simulink model "model_wszystkie_3"  (R2024a)
settings: Solver=ode45  StartTime=0.0  StopTime=60  RelTol=1e-3
InitFcn:
  | a = 0.672; % M + ma/2 + mb, kg
  | b = 0.0051; % (ma/2 + mb)*L, kg*m
  | % c = 0.0021; % (ma/4 + mb)*L^2 + I, kg*m^2
  | g = 9.81;
  | u = 1;
  | 
  | T1 = 0.2;
  | T2 = 0.1;
  | Tf = 0.05;
  | 
  | x1 = 0;
  | x2 = 0;
  | x3 = 0;
  | x4 = 0;
  | x1p = 0;
  | x2p = 0;
  | x3p = 0;
  | x4p = 0;
  | 
  | r = 1;
  | 
  | b0 = 1;
  | A = [0 1 0;
  |      0 0 1;
  |      0 0 0];
  | b_ = [0; b0; 0];
  | c = [1; 0; 0];
  | 
  | % A_CP = [0 1;
  | %        0 0];
  | %
  | % b_CP = [0; 1];
  | %
  | % w_CL = 70;
  | %
  | % k = place(A_CP', b_CP, -w_CL*[1 1.01])';
  | %
  | % k_ESO = 0.9;
  | %
  | % l = place(A',c,-w_CL*k_ESO*[0.99,1,1.01])';
  | 
  | % k_ESO = 10;
  | 
  | % wc_ = 70;
  | % Kx_ = place(A',b_,-wc_*[1 1])';
  | %
  | % k = [5;5];
  | %
  | % w0 = 60;
  | % l = place(A',c,-w0*[0.99,1,1.01])';
  | 
  | %% Liczenie k
  | w_CL = 5;
  | n=2;
  | k = zeros(n,1);
  | for i = 1:n
  |     k(i) = ((factorial(n))/(factorial(n-i+1)*factorial(i-1)))*w_CL^(n-i+1);
  | end
  | 
  | k_r = [k(2); 1];
  | 
  | %% Liczenie l
  | k_ESO = 50;
  | l = zeros(n+1,1);
  | 
  | for i = 1:n+1
  |     l(i) = (factorial(n+1)/(factorial(n-i+1)*factorial(i)))*(k_ESO)^(i);
  | end
  | 
  | % %% PRZYPISANIE POSZCZEGÓLNYCH L:
  | % l1 = l(1);
  | % l2 = l(2);
  | % %% OKREŚLENIE BETY:
  | % B1 = 3 * k_ESO;
  | % B2 = 3 * k_ESO^2;
  | % B3 = k_ESO^3;
  | 
  | %% W ARTYKULE MADONSKI K,L ODPOWIADA L I B W ARTYKULE JIN H.
  | l1 = k(2);
  | l2 = k(1);
  | 
  | B1 = l(1);
  | B2 = l(2);
  | B3 = l(3);
  | 
  | %% WYZNACZENIE PARAMETRÓW:
  | Kc = (B2 * l2 + B3 * l1)/(b0*(B1 * l1 + B2 + l2));
  | tau_i = (B2 * l2 + B3 * l1)/(B3 * l2);
  | tau_d = (B1 * l2 + B2 * l1 + B3)/(B2 * l2 + B3 * l1);
  | wl = sqrt(B1 * l1 + B2 + l2);
  | zeta_l = (B1 + l1)/(2*sqrt(B1 * l1 + B2 + l2));
  | %% Wzmocnienia regulatora CPID:
  | Kp = Kc;
  | Ki = Kc/tau_i;
  | Kd = Kc * tau_d;
  | 
  | %% NOWE NASTAWY PID
  | % Kp = (k(1)*l(1)+k(2)*l(3))/(b0*(k(2)*l(1)+l(2)+k(1)));
  | % Ki = (k(1)*l(3))/(b0*(k(2)*l(1)+l(2)+k(1)));
  | % Kd = (k(1)*l(1)+k(2)*l(2)+l(3))/(b0*(k(2)*l(1)+l(2)+k(1)));
libraries: simulink x4, slpidlib x1
settings Model: Creator=kubat  LastModifiedBy=kubat
settings OptimizationCC: ReuseModelBlockBuffer=off
settings RTWCC: GPUComputeCapability=3.5

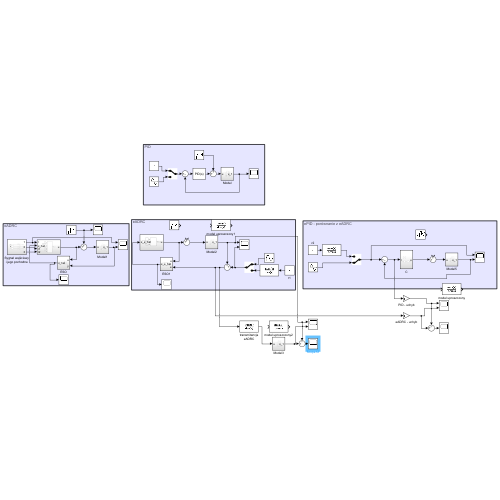
[thumbnail: Simulink's stored preview of the top-level diagram]
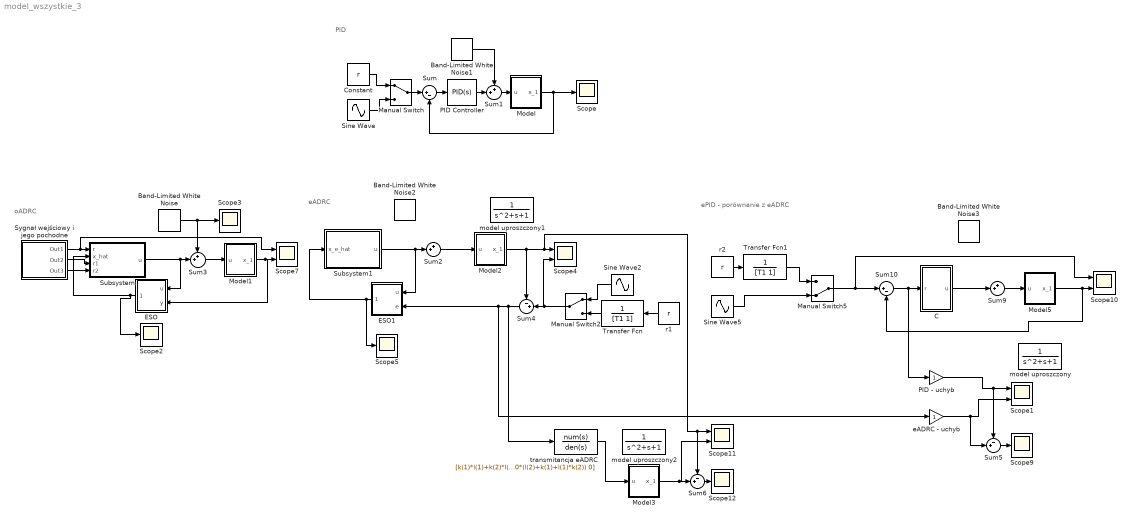
== system model_wszystkie_3 ==
  note: eADRC
  note: oADRC
  note: PID
  note: ePID - porównanie z eADRC
  Band-Limited White Noise{,1..3} (4 alike) : simulink/Sources/Band-Limited White Noise  Cov=[0.001]  Ts=0.01  seed=[23341]
  C : Subsystem
  Constant : Constant  Value=r
  ESO : Subsystem
  ESO1 : Subsystem
  Manual Switch : ManualSwitch
  Manual Switch2 : ManualSwitch
  Manual Switch5 : ManualSwitch  CurrentSetting=0
  Model : Subsystem
  Model1 : Subsystem
  Model2 : Subsystem
  Model3 : Subsystem
  Model5 : Subsystem
  PID - uchyb : Gain
  PID Controller : slpidlib/PID Controller  Controller=PID  Form=Parallel  TimeDomain=Continuous-time  UseExternalTs=off  SampleTime=-1  IntegratorMethod=Forward Euler  FilterMethod=Forward Euler  ControllerParametersSource=internal  P=0.00659119654590323  I=2.38451819654017e-05  UseKiTs=off  D=0.404807783978182  UseExternalDerivativeSource=off  N=70.8689683200542  UseFilter=on  TunerSelectOption=Transfer Function Based (PID Tuner App)  InitialConditionSource=internal  InitialConditionForIntegrator=0  InitialConditionForFilter=0  DifferentiatorICPrevScaledInput=0  ExternalReset=none  TrackingMode=off  Kt=1  LimitOutput=off  SatLimitsSource=internal  UpperSaturationLimit=inf  LowerSaturationLimit=-inf  LinearizeAsGain=on  AntiWindupMode=none  Kb=1  LimitIntegrator=off  UpperIntegratorSaturationLimit=inf  LowerIntegratorSaturationLimit=-inf  POutMin=[]  POutMax=[]  IOutMin=[]  IOutMax=[]  DOutMin=[]  DOutMax=[]  NOutMin=[]  NOutMax=[]  SumOutMin=[]  SumOutMax=[]  SaturationOutMin=[]  SaturationOutMax=[]  PParamMin=[]  PParamMax=[]  IParamMin=[]  IParamMax=[]  DParamMin=[]  DParamMax=[]  NParamMin=[]  NParamMax=[]  KbParamMin=[]  KbParamMax=[]  KtParamMin=[]  KtParamMax=[]  KbOutMin=[]  KbOutMax=[]  KtOutMin=[]  KtOutMax=[]  IntegratorOutMin=[]  IntegratorOutMax=[]  FilterOutMin=[]  FilterOutMax=[]  SumI1OutMin=[]  SumI1OutMax=[]  SumI2OutMin=[]  SumI2OutMax=[]  SumI3OutMin=[]  SumI3OutMax=[]  SumI4OutMin=[]  SumI4OutMax=[]  SumDOutMin=[]  SumDOutMax=[]  DifferentiatorOutMin=[]  DifferentiatorOutMax=[]  FilterDiffOutCoefMin=[]  FilterDiffOutCoefMax=[]  ReciprocalOutMin=[]  ReciprocalOutMax=[]  SumDenOutMin=[]  SumDenOutMax=[]  SumNumOutMin=[]  SumNumOutMax=[]  DivideOutMin=[]  DivideOutMax=[]  UdiffTsProdOutMin=[]  UdiffTsProdOutMax=[]  NTsProdOutMin=[]  NTsProdOutMax=[]  UintegralTsProdOutMin=[]  UintegralTsProdOutMax=[]  UngainTsProdOutMin=[]  UngainTsProdOutMax=[]  ClampingZeroOutDataTypeStr=Inherit: Inherit via back propagation  ClampingZeroOutMin=[]  ClampingZeroOutMax=[]  FilterDenConstantOutDataTypeStr=Inherit: Inherit via back propagation  FilterDenConstantOutMin=[]  FilterDenConstantOutMax=[]  PCopyOutDataTypeStr=Inherit: Inherit via back propagation  PCopyOutMin=[]  PCopyOutMax=[]  NCopyOutDataTypeStr=Inherit: Inherit via back propagation  NCopyOutMin=[]  NCopyOutMax=[]  IntegratorContinuousStateAttributes=''  IntegratorStateMustResolveToSignalObject=off  IntegratorRTWStateStorageClass=Auto  FilterContinuousStateAttributes=''  FilterStateMustResolveToSignalObject=off  FilterRTWStateStorageClass=Auto  ParallelPVariant=InternalParameters  IdealPVariant=Disabled  IVariant=InternalParameters  DVariant=InternalParameters  IntegratorVariant=Continuous  SatVariant=Disabled  AWVariant=Passthrough  PCopyVariant=Disabled  TRVariant=Disabled  FdbkBlocksVariant=Forward  IdealPFdbkVariant=Disabled  SatFdbkVariant=Disabled  DerivativeFilterVariant=ContFilter  NVariant=InternalParameters  NCopyVariant=Disabled  FilterICVariant=InternalICsFilter  IntegratorICVariant=InternalICs  ExternalResetVariant=Disabled  TRSumVariant=Passthrough  SumFdbkVariant=Disabled  SumVariant=Sum_PID  TsampFilterVariant=InternalTs  TsampNgainVariant=Passthrough  TsampIntegralVariant=Disabled_SignalSpec  ExternalSaturationOutDataTypeStr=Inherit: Same as second input  DerivativeSourceVariant=ErrorSignal
  Scope{,2..3,5,9,12} (6 alike) : Scope
  Scope{1,4,7,10..11} (5 alike) : Scope  NumInputPorts=2
  Sine Wave : Sin  Amplitude=u  SampleTime=0
  Sine Wave2 : Sin  Amplitude=u  SampleTime=0
  Sine Wave5 : Sin  Amplitude=u  SampleTime=0
  Subsystem : Subsystem
  Subsystem1 : Subsystem
  Sum : Sum  Inputs=|+-
  Sum{1..3,9} (4 alike) : Sum  Inputs=++|
  Sum10 : Sum  Inputs=|+-
  Sum4 : Sum  Inputs=-+|
  Sum5 : Sum  Inputs=-+|
  Sum6 : Sum  Inputs=-+|
  Sygnał wejściowy i jego pochodne : Subsystem
  Transfer Fcn : TransferFcn  Denominator=[T1 1]
  Transfer Fcn1 : TransferFcn  Denominator=[T1 1]
  eADRC - uchyb : Gain
  model uproszczony : TransferFcn  Denominator=[1 1 1]
  model uproszczony1 : TransferFcn  Denominator=[1 1 1]
  model uproszczony2 : TransferFcn  Denominator=[1 1 1]
  r1 : Constant  Value=r
  r2 : Constant  Value=r
  transmitancja eADRC : TransferFcn  Numerator=[k(1)*l(1)+k(2)*l(2)+l(3) k(1)*l(2)+k(2)*l(3) k(1)*l(3)]  Denominator=[b0 b0*(k(2)+l(1)) b0*(l(2)+k(1)+l(1)*k(2)) 0]
  wires:
  Model/1(x_1) -> Scope/1, Sum/2
  Sum/1 -> PID Controller/1
  Manual Switch/1 -> Sum/1
  Constant/1 -> Manual Switch/1
  Sine Wave/1 -> Manual Switch/2
  Model1/1(x_1) -> ESO/2(y), Scope7/2
  Sum3/1 -> Model1/1(u)
  Subsystem/1(u) -> ESO/1(u), Sum3/2
  ESO/1(x_hat) -> Scope2/1, Subsystem/2(x_hat)
  Band-Limited White Noise/1 -> Sum3/1, Scope3/1
  PID Controller/1 -> Sum1/2
  Sum1/1 -> Model/1(u)
  Band-Limited White Noise1/1 -> Sum1/1
  ESO1/1(x_e_hat) -> Subsystem1/1(x_e_hat), Scope5/1
  Subsystem1/1(u) -> ESO1/1(u), Sum2/2
  Sum4/1 -> transmitancja eADRC/1, eADRC - uchyb/1, ESO1/2(e)
  Sine Wave2/1 -> Manual Switch2/1
  Manual Switch2/1 -> Scope4/2, Sum4/2
  Transfer Fcn/1 -> Manual Switch2/2
  r1/1 -> Transfer Fcn/1
  Sygnał wejściowy i jego pochodne/1(Out1) -> Scope7/1, Subsystem/1(r)
  Sygnał wejściowy i jego pochodne/2(Out2) -> Subsystem/3(r1)
  Sygnał wejściowy i jego pochodne/3(Out3) -> Subsystem/4(r2)
  C/1(u) -> Sum9/2
  Sum10/1 -> PID - uchyb/1, C/1(r)
  Sine Wave5/1 -> Manual Switch5/2
  Manual Switch5/1 -> Scope10/1, Sum10/1
  Transfer Fcn1/1 -> Manual Switch5/1
  r2/1 -> Transfer Fcn1/1
  PID - uchyb/1 -> Sum5/1, Scope1/1
  eADRC - uchyb/1 -> Sum5/2, Scope1/2
  Sum5/1 -> Scope9/1
  Sum9/1 -> Model5/1(u)
  Model5/1(x_1) -> Sum10/2, Scope10/2
  Sum2/1 -> Model2/1(u)
  Model2/1(x_1) -> Scope11/1, Sum6/1, Scope4/1, Sum4/1
  transmitancja eADRC/1 -> Model3/1(u)
  Model3/1(x_1) -> Scope11/2, Sum6/2
  Sum6/1 -> Scope12/1

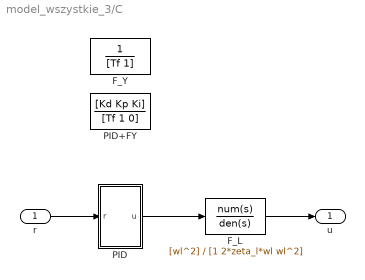
== system model_wszystkie_3/C ==
  r : Inport
  F_L : TransferFcn  Numerator=[wl^2]  Denominator=[1 2*zeta_l*wl wl^2]
  F_Y : TransferFcn  Denominator=[Tf 1]
  PID : Subsystem
  PID+FY : TransferFcn  Numerator=[Kd Kp Ki]  Denominator=[Tf 1 0]
  u : Outport
  wires:
  PID/1(u) -> F_L/1
  r/1 -> PID/1(r)
  F_L/1 -> u/1

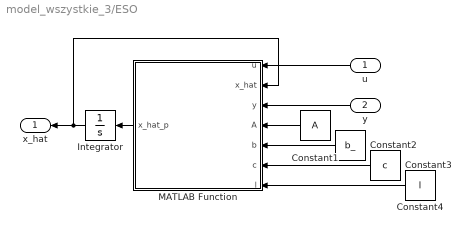
== system model_wszystkie_3/ESO ==
  u : Inport
  y : Inport  Port=2
  Constant1 : Constant  Value=A
  Constant2 : Constant  Value=b_
  Constant3 : Constant  Value=c
  Constant4 : Constant  Value=l
  Integrator : Integrator
  MATLAB Function : MATLAB Function  TreatAsAtomicUnit=on
  x_hat : Outport
  wires:
  Constant3/1 -> MATLAB Function/6(c)
  Integrator/1 -> x_hat/1, MATLAB Function/2(x_hat)
  MATLAB Function/1(x_hat_p) -> Integrator/1
  Constant2/1 -> MATLAB Function/5(b)
  y/1 -> MATLAB Function/3(y)
  Constant1/1 -> MATLAB Function/4(A)
  Constant4/1 -> MATLAB Function/7(l)
  u/1 -> MATLAB Function/1(u)

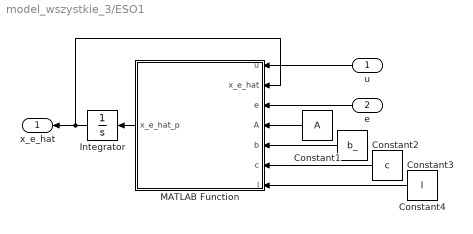
== system model_wszystkie_3/ESO1 ==
  u : Inport
  e : Inport  Port=2
  Constant1 : Constant  Value=A
  Constant2 : Constant  Value=b_
  Constant3 : Constant  Value=c
  Constant4 : Constant  Value=l
  Integrator : Integrator
  MATLAB Function : MATLAB Function  TreatAsAtomicUnit=on
  x_e_hat : Outport
  wires:
  Constant3/1 -> MATLAB Function/6(c)
  Integrator/1 -> x_e_hat/1, MATLAB Function/2(x_e_hat)
  MATLAB Function/1(x_e_hat_p) -> Integrator/1
  Constant2/1 -> MATLAB Function/5(b)
  e/1 -> MATLAB Function/3(e)
  Constant1/1 -> MATLAB Function/4(A)
  Constant4/1 -> MATLAB Function/7(l)
  u/1 -> MATLAB Function/1(u)

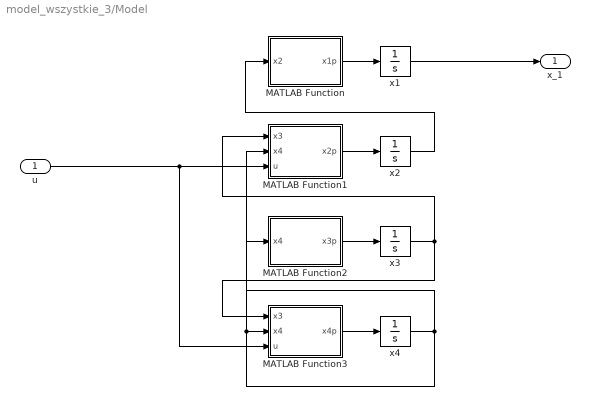
== system model_wszystkie_3/Model ==
  u : Inport
  MATLAB Function : MATLAB Function  TreatAsAtomicUnit=on
  MATLAB Function1 : MATLAB Function  TreatAsAtomicUnit=on
  MATLAB Function2 : MATLAB Function  TreatAsAtomicUnit=on
  MATLAB Function3 : MATLAB Function  TreatAsAtomicUnit=on
  x{1..4} (4 alike) : Integrator
  x_1 : Outport
  wires:
  u/1 -> MATLAB Function3/3(u), MATLAB Function1/3(u)
  x4/1 -> MATLAB Function3/2(x4), MATLAB Function1/2(x4), MATLAB Function2/1(x4)
  MATLAB Function/1(x1p) -> x1/1
  x3/1 -> MATLAB Function1/1(x3), MATLAB Function3/1(x3)
  x2/1 -> MATLAB Function/1(x2)
  MATLAB Function2/1(x3p) -> x3/1
  MATLAB Function1/1(x2p) -> x2/1
  MATLAB Function3/1(x4p) -> x4/1
  x1/1 -> x_1/1

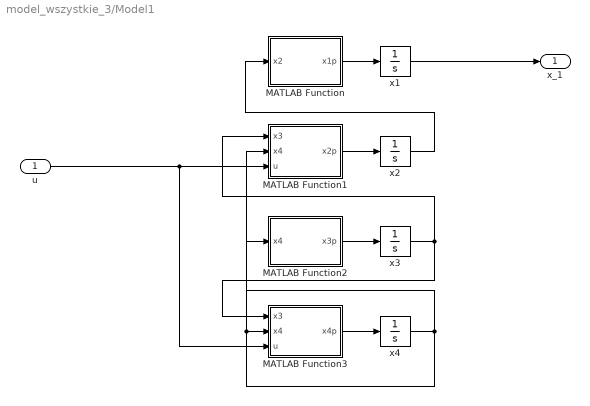
== system model_wszystkie_3/Model1 ==
  u : Inport
  MATLAB Function : MATLAB Function  TreatAsAtomicUnit=on
  MATLAB Function1 : MATLAB Function  TreatAsAtomicUnit=on
  MATLAB Function2 : MATLAB Function  TreatAsAtomicUnit=on
  MATLAB Function3 : MATLAB Function  TreatAsAtomicUnit=on
  x{1..4} (4 alike) : Integrator
  x_1 : Outport
  wires:
  u/1 -> MATLAB Function3/3(u), MATLAB Function1/3(u)
  x4/1 -> MATLAB Function3/2(x4), MATLAB Function1/2(x4), MATLAB Function2/1(x4)
  MATLAB Function/1(x1p) -> x1/1
  x3/1 -> MATLAB Function1/1(x3), MATLAB Function3/1(x3)
  x2/1 -> MATLAB Function/1(x2)
  MATLAB Function2/1(x3p) -> x3/1
  MATLAB Function1/1(x2p) -> x2/1
  MATLAB Function3/1(x4p) -> x4/1
  x1/1 -> x_1/1

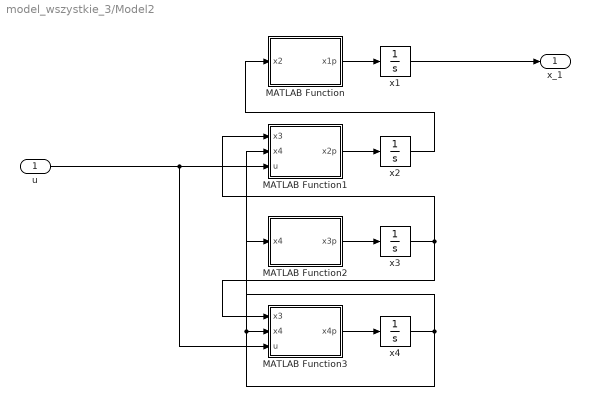
== system model_wszystkie_3/Model2 ==
  u : Inport
  MATLAB Function : MATLAB Function  TreatAsAtomicUnit=on
  MATLAB Function1 : MATLAB Function  TreatAsAtomicUnit=on
  MATLAB Function2 : MATLAB Function  TreatAsAtomicUnit=on
  MATLAB Function3 : MATLAB Function  TreatAsAtomicUnit=on
  x{1..4} (4 alike) : Integrator
  x_1 : Outport
  wires:
  u/1 -> MATLAB Function3/3(u), MATLAB Function1/3(u)
  x4/1 -> MATLAB Function2/1(x4), MATLAB Function3/2(x4), MATLAB Function1/2(x4)
  MATLAB Function/1(x1p) -> x1/1
  x3/1 -> MATLAB Function1/1(x3), MATLAB Function3/1(x3)
  x2/1 -> MATLAB Function/1(x2)
  MATLAB Function2/1(x3p) -> x3/1
  MATLAB Function1/1(x2p) -> x2/1
  MATLAB Function3/1(x4p) -> x4/1
  x1/1 -> x_1/1

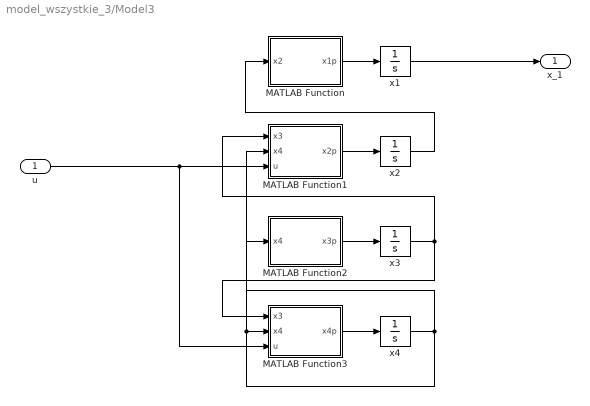
== system model_wszystkie_3/Model3 ==
  u : Inport
  MATLAB Function : MATLAB Function  TreatAsAtomicUnit=on
  MATLAB Function1 : MATLAB Function  TreatAsAtomicUnit=on
  MATLAB Function2 : MATLAB Function  TreatAsAtomicUnit=on
  MATLAB Function3 : MATLAB Function  TreatAsAtomicUnit=on
  x{1..4} (4 alike) : Integrator
  x_1 : Outport
  wires:
  u/1 -> MATLAB Function3/3(u), MATLAB Function1/3(u)
  x4/1 -> MATLAB Function3/2(x4), MATLAB Function1/2(x4), MATLAB Function2/1(x4)
  MATLAB Function/1(x1p) -> x1/1
  x3/1 -> MATLAB Function1/1(x3), MATLAB Function3/1(x3)
  x2/1 -> MATLAB Function/1(x2)
  MATLAB Function2/1(x3p) -> x3/1
  MATLAB Function1/1(x2p) -> x2/1
  MATLAB Function3/1(x4p) -> x4/1
  x1/1 -> x_1/1

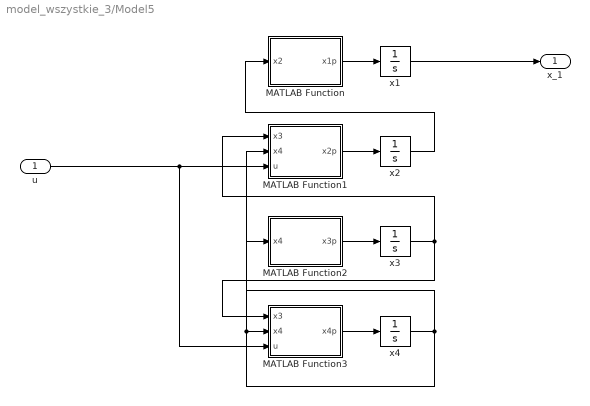
== system model_wszystkie_3/Model5 ==
  u : Inport
  MATLAB Function : MATLAB Function  TreatAsAtomicUnit=on
  MATLAB Function1 : MATLAB Function  TreatAsAtomicUnit=on
  MATLAB Function2 : MATLAB Function  TreatAsAtomicUnit=on
  MATLAB Function3 : MATLAB Function  TreatAsAtomicUnit=on
  x{1..4} (4 alike) : Integrator
  x_1 : Outport
  wires:
  u/1 -> MATLAB Function3/3(u), MATLAB Function1/3(u)
  x4/1 -> MATLAB Function3/2(x4), MATLAB Function1/2(x4), MATLAB Function2/1(x4)
  MATLAB Function/1(x1p) -> x1/1
  x3/1 -> MATLAB Function1/1(x3), MATLAB Function3/1(x3)
  x2/1 -> MATLAB Function/1(x2)
  MATLAB Function2/1(x3p) -> x3/1
  MATLAB Function1/1(x2p) -> x2/1
  MATLAB Function3/1(x4p) -> x4/1
  x1/1 -> x_1/1

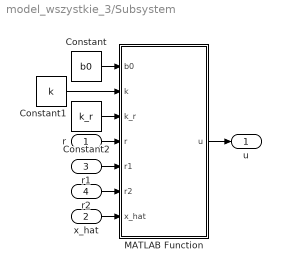
== system model_wszystkie_3/Subsystem ==
  r : Inport
  x_hat : Inport  Port=2
  r1 : Inport  Port=3
  r2 : Inport  Port=4
  Constant : Constant  Value=b0
  Constant1 : Constant  Value=k
  Constant2 : Constant  Value=k_r
  MATLAB Function : MATLAB Function  TreatAsAtomicUnit=on
  u : Outport
  wires:
  Constant/1 -> MATLAB Function/1(b0)
  Constant1/1 -> MATLAB Function/2(k)
  r/1 -> MATLAB Function/4(r)
  x_hat/1 -> MATLAB Function/7(x_hat)
  MATLAB Function/1(u) -> u/1
  r1/1 -> MATLAB Function/5(r1)
  r2/1 -> MATLAB Function/6(r2)
  Constant2/1 -> MATLAB Function/3(k_r)

== system model_wszystkie_3/Subsystem1 ==
  x_e_hat : Inport
  Constant : Constant  Value=b0
  Constant1 : Constant  Value=k
  MATLAB Function : MATLAB Function  TreatAsAtomicUnit=on
  u : Outport
  wires:
  Constant/1 -> MATLAB Function/1(b0)
  Constant1/1 -> MATLAB Function/2(k)
  x_e_hat/1 -> MATLAB Function/3(x_e_hat)
  MATLAB Function/1(u) -> u/1

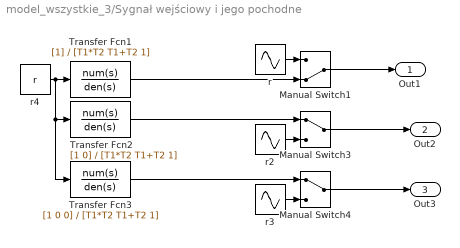
== system model_wszystkie_3/Sygnał wejściowy i jego pochodne ==
  Manual Switch1 : ManualSwitch  CurrentSetting=0
  Manual Switch3 : ManualSwitch
  Manual Switch4 : ManualSwitch
  Transfer Fcn1 : TransferFcn  Denominator=[T1*T2 T1+T2 1]
  Transfer Fcn2 : TransferFcn  Numerator=[1 0]  Denominator=[T1*T2 T1+T2 1]
  Transfer Fcn3 : TransferFcn  Numerator=[1 0 0]  Denominator=[T1*T2 T1+T2 1]
  r : Sin  Amplitude=u  SampleTime=0
  r2 : Sin  Amplitude=u  Phase=pi/2  SampleTime=0
  r3 : Sin  Amplitude=-u  SampleTime=0
  r4 : Constant  Value=r
  Out1 : Outport
  Out2 : Outport  Port=2
  Out3 : Outport  Port=3
  wires:
  Transfer Fcn1/1 -> Manual Switch1/2
  r2/1 -> Manual Switch3/2
  r/1 -> Manual Switch1/1
  Manual Switch1/1 -> Out1/1
  r3/1 -> Manual Switch4/2
  Transfer Fcn2/1 -> Manual Switch3/1
  r4/1 -> Transfer Fcn3/1, Transfer Fcn2/1, Transfer Fcn1/1
  Transfer Fcn3/1 -> Manual Switch4/1
  Manual Switch4/1 -> Out3/1
  Manual Switch3/1 -> Out2/1

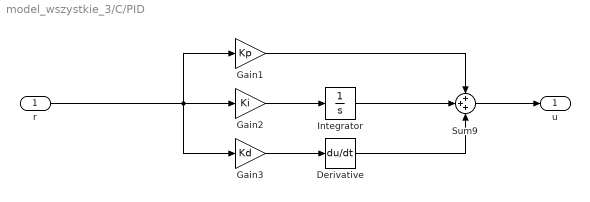
== system model_wszystkie_3/C/PID ==
  r : Inport
  Derivative : Derivative
  Gain1 : Gain  Gain=Kp
  Gain2 : Gain  Gain=Ki
  Gain3 : Gain  Gain=Kd
  Integrator : Integrator
  Sum9 : Sum  Inputs=+++
  u : Outport
  wires:
  Gain1/1 -> Sum9/1
  r/1 -> Gain3/1, Gain2/1, Gain1/1
  Gain2/1 -> Integrator/1
  Gain3/1 -> Derivative/1
  Sum9/1 -> u/1
  Derivative/1 -> Sum9/3
  Integrator/1 -> Sum9/2

== matlab function model_wszystkie_3/ESO1/MATLAB Function ==
  data: u input; x_e_hat_p output; x_e_hat input; e input; A input; b input; c input; l input
function x_e_hat_p = fcn(u, x_e_hat, e, A, b, c, l)
c = c.';
pom1 = c*x_e_hat;
pom2 = e - pom1;

x_e_hat_p1 = A*x_e_hat-b*u+l*pom2;
x_e_hat_p = x_e_hat_p1(:,1);

== matlab function model_wszystkie_3/Model2/MATLAB Function ==
  data: x2 input; x1p output
function x1p = fcn(x2)

x1p = x2;

== matlab function model_wszystkie_3/Model2/MATLAB Function1 ==
  data: x3 input; x2p output; x4 input; u input
function x2p = fcn(x3, x4,u)
g = 9.81;
x2p = ((0.0031*u)/(0.0021-0.000038*cos(x3)^2))-(0.000016*sin(x3)*x4^2+0.000038*g*sin(x3)*cos(x3))/(0.0021-0.000038*cos(x3)^2);

== matlab function model_wszystkie_3/Model/MATLAB Function1 ==
  data: x3 input; x2p output; x4 input; u input
function x2p = fcn(x3, x4,u)
g = 9.81;
x2p = ((0.0031*u)/(0.0021-0.000038*cos(x3)^2))-(0.000016*sin(x3)*x4^2+0.000038*g*sin(x3)*cos(x3))/(0.0021-0.000038*cos(x3)^2);

== matlab function model_wszystkie_3/Model2/MATLAB Function2 ==
  data: x4 input; x3p output
function x3p = fcn(x4)

x3p = x4;

== matlab function model_wszystkie_3/Model2/MATLAB Function3 ==
  data: x3 input; x4 input; x4p output; u input
function x4p = fcn(x3,x4,u)
g = 9.81;
x4p = ((-0.0076*cos(x3)*u)/(0.0021-0.000038*cos(x3)^2))+(((-0.000038*sin(x3)*cos(x3)*x4^2) + 0.0051*g*sin(x3))/(0.0021-0.000038*cos(x3)^2));

== matlab function model_wszystkie_3/Subsystem1/MATLAB Function ==
  data: b0 input; u output; k input; x_e_hat input
function u = fcn(b0, k, x_e_hat)

k = k';
kpom = [k, 1];
b0_1 = 1/b0;
u = b0_1*(kpom*x_e_hat);

== matlab function model_wszystkie_3/Model3/MATLAB Function ==
  data: x2 input; x1p output
function x1p = fcn(x2)

x1p = x2;

== matlab function model_wszystkie_3/Model3/MATLAB Function1 ==
  data: x3 input; x2p output; x4 input; u input
function x2p = fcn(x3, x4,u)
g = 9.81;
x2p = ((0.0031*u)/(0.0021-0.000038*cos(x3)^2))-(0.000016*sin(x3)*x4^2+0.000038*g*sin(x3)*cos(x3))/(0.0021-0.000038*cos(x3)^2);

== matlab function model_wszystkie_3/Model3/MATLAB Function2 ==
  data: x4 input; x3p output
function x3p = fcn(x4)

x3p = x4;

== matlab function model_wszystkie_3/Model3/MATLAB Function3 ==
  data: x3 input; x4 input; x4p output; u input
function x4p = fcn(x3,x4,u)
g = 9.81;
x4p = ((-0.0076*cos(x3)*u)/(0.0021-0.000038*cos(x3)^2))+(((-0.000038*sin(x3)*cos(x3)*x4^2) + 0.0051*g*sin(x3))/(0.0021-0.000038*cos(x3)^2));

== matlab function model_wszystkie_3/Model5/MATLAB Function ==
  data: x2 input; x1p output
function x1p = fcn(x2)

x1p = x2;

== matlab function model_wszystkie_3/Model5/MATLAB Function1 ==
  data: x3 input; x2p output; x4 input; u input
function x2p = fcn(x3, x4,u)
g = 9.81;
x2p = ((0.0031*u)/(0.0021-0.000038*cos(x3)^2))-(0.000016*sin(x3)*x4^2+0.000038*g*sin(x3)*cos(x3))/(0.0021-0.000038*cos(x3)^2);

== matlab function model_wszystkie_3/Model5/MATLAB Function2 ==
  data: x4 input; x3p output
function x3p = fcn(x4)

x3p = x4;

== matlab function model_wszystkie_3/Model5/MATLAB Function3 ==
  data: x3 input; x4 input; x4p output; u input
function x4p = fcn(x3,x4,u)
g = 9.81;
x4p = ((-0.0076*cos(x3)*u)/(0.0021-0.000038*cos(x3)^2))+(((-0.000038*sin(x3)*cos(x3)*x4^2) + 0.0051*g*sin(x3))/(0.0021-0.000038*cos(x3)^2));

== matlab function model_wszystkie_3/Model/MATLAB Function ==
  data: x2 input; x1p output
function x1p = fcn(x2)

x1p = x2;

== matlab function model_wszystkie_3/Model/MATLAB Function2 ==
  data: x4 input; x3p output
function x3p = fcn(x4)

x3p = x4;

== matlab function model_wszystkie_3/Model/MATLAB Function3 ==
  data: x3 input; x4 input; x4p output; u input
function x4p = fcn(x3,x4,u)
g = 9.81;
x4p = ((-0.0076*cos(x3)*u)/(0.0021-0.000038*cos(x3)^2))+(((-0.000038*sin(x3)*cos(x3)*x4^2) + 0.0051*g*sin(x3))/(0.0021-0.000038*cos(x3)^2));

== matlab function model_wszystkie_3/Model1/MATLAB Function ==
  data: x2 input; x1p output
function x1p = fcn(x2)

x1p = x2;

== matlab function model_wszystkie_3/Model1/MATLAB Function1 ==
  data: x3 input; x2p output; x4 input; u input
function x2p = fcn(x3, x4,u)
g = 9.81;
x2p = ((0.0031*u)/(0.0021-0.000038*cos(x3)^2))-(0.000016*sin(x3)*x4^2+0.000038*g*sin(x3)*cos(x3))/(0.0021-0.000038*cos(x3)^2);

== matlab function model_wszystkie_3/Model1/MATLAB Function2 ==
  data: x4 input; x3p output
function x3p = fcn(x4)

x3p = x4;

== matlab function model_wszystkie_3/Model1/MATLAB Function3 ==
  data: x3 input; x4 input; x4p output; u input
function x4p = fcn(x3,x4,u)
g = 9.81;
x4p = ((-0.0076*cos(x3)*u)/(0.0021-0.000038*cos(x3)^2))+(((-0.000038*sin(x3)*cos(x3)*x4^2) + 0.0051*g*sin(x3))/(0.0021-0.000038*cos(x3)^2));

== matlab function model_wszystkie_3/ESO/MATLAB Function ==
  data: u input; x_hat_p output; x_hat input; y input; A input; b input; c input; l input
function x_hat_p = fcn(u, x_hat, y, A, b, c, l)
c = c.';
pom1 = c*x_hat;
pom2 = y - pom1;

x_hat_p1 = A*x_hat+b*u+l*pom2;
x_hat_p = x_hat_p1(:,1);

== matlab function model_wszystkie_3/Subsystem/MATLAB Function ==
  data: b0 input; u output; k input; k_r input; r input; r1 input; r2 input; x_hat input
function u = fcn(b0, k, k_r, r, r1, r2, x_hat)


kpom = [k; 1].';
r_d = [r1; r2];
k_r = k_r';
b0_1 = 1/b0;

u = b0_1*(k(1)*r+k_r*r_d-(kpom*x_hat));
